simulink model "tilting_holocopter_approach"  (R2023b)
settings: Solver=VariableStepAuto  StartTime=0.0  StopTime=tot_time  RelTol=1e-3
InitFcn:
  | addpath('TRAJECTORIES\');
  | square_tilting
  | %circular_tilting
StartFcn:
  | %% Setup Video e Timer
  | videoFile = 'Holocopter_quad.avi';
  | %videoFile = 'Holocopter_circ.avi';
  | videoObj = VideoWriter(videoFile);
  | videoObj.FrameRate = 30;
  | open(videoObj);
  | assignin('base','videoObj',videoObj);
  | 
  | 
  | t = timer('ExecutionMode','fixedSpacing','Period',0.05,'StartDelay',2,...
  |           'TimerFcn',@(~,~) captureFrame(findall(0,'Type','figure','Name','UAV Animation'), videoObj));
  | start(t);
  | 
  | 
  | assignin('base','videoTimer',t);
StopFcn:
  | % Default graphics settings
  | set(0, 'DefaultTextInterpreter', 'latex')
  | set(0, 'DefaultLegendInterpreter', 'latex')
  | set(0, 'DefaultAxesTickLabelInterpreter', 'latex')
  | lw = 2;
  | plot_errors = figure('Renderer', 'painters', 'Position', [10 10 900 650]);
  | subplot(3,1,1)
  | plot(out.err_p.time, out.err_p.signals.values(1,:), 'k-', 'Linewidth', lw ,'Color', [0.2, 0.2, 0.2]);
  | hold on
  | plot(out.err_p.time, out.err_p.signals.values(2,:), 'k-', 'Linewidth', lw ,'Color', [1, 0, 0]);
  | hold on
  | plot(out.err_p.time, out.err_p.signals.values(3,:), 'k-', 'Linewidth', lw ,'Color', [0, 0, 1]);
  | legend({'x-axis', 'y-axis', 'z-axis'}, ...
  |        'Location', 'southeast', ...
  |        'Orientation', 'vertical', ...
  |        'FontSize', 12);
  | %xlabel('Time [s]')
  | ylabel('$e_p$ [m]')
  | set(gca, 'FontSize',18);
  | %Grid
  | grid on
  | box on
  | %----------------------------------------------------------
  | subplot(3,1,2)
  | plot(out.dot_err_p.time, out.dot_err_p.signals.values(1,:), 'k-', 'Linewidth', lw ,'Color', [0.2, 0.2, 0.2]);
  | hold on
  | plot(out.dot_err_p.time, out.dot_err_p.signals.values(2,:), 'k-', 'Linewidth', lw ,'Color', [1, 0, 0]);
  | hold on
  | plot(out.dot_err_p.time, out.dot_err_p.signals.values(3,:), 'k-', 'Linewidth', lw ,'Color', [0, 0, 1]);
  | legend({'x-axis', 'y-axis', 'z-axis'}, ...
  |        'Location', 'southeast', ...
  |        'Orientation', 'vertical', ...
  |        'FontSize', 12);
  | 
  | ylabel('$\dot{e}_p$ [m/s]')
  | set(gca, 'FontSize',18);
  | %Grid
  | grid on
  | box on
  | subplot(3,1,3)
  | plot(out.ddot_err_p.time, out.dot_err_p.signals.values(1,:), 'k-', 'Linewidth', lw ,'Color', [0.2, 0.2, 0.2]);
  | hold on
  | plot(out.ddot_err_p.time, out.dot_err_p.signals.values(2,:), 'k-', 'Linewidth', lw ,'Color', [1, 0, 0]);
  | hold on
  | plot(out.ddot_err_p.time, out.dot_err_p.signals.values(3,:), 'k-', 'Linewidth', lw ,'Color', [0, 0, 1]);
  | legend({'x-axis', 'y-axis', 'z-axis'}, ...
  |        'Location', 'southeast', ...
  |        'Orientation', 'vertical', ...
  |        'FontSize', 12);
  | xlabel('Time [s]')
  | ylabel('$\ddot{e}_p$ [m/$s^2$]')
  | set(gca, 'FontSize',18);
  | %Grid
  | grid on
  | box on
  | %Options
  | set(gcf,'color','w');
  | set(plot_errors, 'MenuBar', 'none', 'ToolBar', 'none');
  | exportgraphics(plot_errors, 'Tilting_holocopter_lin_err.pdf');
  | %--------------------------------------------------
  | plot_errors_or = figure('Renderer', 'painters', 'Position', [10 10 900 650]);
  | subplot(3,1,1)
  | plot(out.eR.time, out.eR.signals.values(1,:), 'k-', 'Linewidth', lw ,'Color', [0.2, 0.2, 0.2]);
  | hold on
  | plot(out.eR.time, out.eR.signals.values(2,:), 'k-', 'Linewidth', lw ,'Color', [1, 0, 0]);
  | hold on
  | plot(out.eR.time, out.eR.signals.values(3,:), 'k-', 'Linewidth', lw ,'Color', [0, 0, 1]);
  | legend({'x-axis', 'y-axis', 'z-axis'}, ...
  |        'Location', 'northeast', ...
  |        'Orientation', 'vertical', ...
  |        'FontSize', 10);
  | ylabel('$e_R$ [rad]')
  | set(gca, 'FontSize',18);
  | %Grid
  | grid on
  | box on
  | %----------------------------------------------------------
  | subplot(3,1,2)
  | plot(out.ew.time, out.ew.signals.values(1,:), 'k-', 'Linewidth', lw ,'Color', [0.2, 0.2, 0.2]);
  | hold on
  | plot(out.ew.time, out.ew.signals.values(2,:), 'k-', 'Linewidth', lw ,'Color', [1, 0, 0]);
  | hold on
  | plot(out.ew.time, out.ew.signals.values(3,:), 'k-', 'Linewidth', lw ,'Color', [0, 0, 1]);
  | legend({'x-axis', 'y-axis', 'z-axis'}, ...
  |        'Location', 'southeast', ...
  |        'Orientation', 'vertical', ...
  |        'FontSize', 10);
  | 
  | ylabel('$e_\omega$ [rad/s]')
  | set(gca, 'FontSize',18);
  | %Grid
  | grid on
  | box on
  | subplot(3,1,3)
  | plot(out.ea.time, out.ea.signals.values(1,:), 'k-', 'Linewidth', lw ,'Color', [0.2, 0.2, 0.2]);
  | hold on
  | plot(out.ea.time, out.ea.signals.values(2,:), 'k-', 'Linewidth', lw ,'Color', [1, 0, 0]);
  | hold on
  | plot(out.ea.time, out.ea.signals.values(3,:), 'k-', 'Linewidth', lw ,'Color', [0, 0, 1]);
  | legend({'x-axis', 'y-axis', 'z-axis'}, ...
  |        'Location', 'northeast', ...
  |        'Orientation', 'vertical', ...
  |        'FontSize', 8);
  | ylabel('$e_a$ [rad/$s^2$]')
  | xlabel('Time [s]')
  | set(gca, 'FontSize',18);
  | %Grid
  | grid on
  | box on
  | %Options
  | set(gcf,'color','w');
  | set(plot_errors_or, 'MenuBar', 'none', 'ToolBar', 'none');
  | exportgraphics(plot_errors_or, 'Tilting_holocopter_or_err.pdf');
  | %---------------------------------------------------------------------
  | 
  | 
  | 
  | %---------------------------------------------------------------------
  | 
  | 
  | videoObj = evalin('base','videoObj');
  | t = evalin('base','videoTimer');
  | 
  | 
  | stop(t);
  | delete(t);
  | close(videoObj);
  | 
  | 
  | clear videoObj videoTimer
  | disp('Saved Video UAV');
values from neighbouring files (symbols this model uses):
  cf = 1.65776*10^(-5)    (= 1.65776e-05)    [myConstraintsFcn.m]
  cm = 2.1792*10^(-7)    (= 2.1792e-07)    [myConstraintsFcn.m]
  l = 0.45    [myConstraintsFcn.m]
undefined symbols (not defined in the file or in its folder): Ib, lin_vel_0, mass, pos_0, Ts, w_bb_0
libraries: robotcorelib x1, matrix_library x1, uavutilslib x1
settings Model: Creator=fabioruggiero  LastModifiedBy=laura
settings ModelReferenceCC: EnableRefExpFcnMdlSchedulingChecks=on

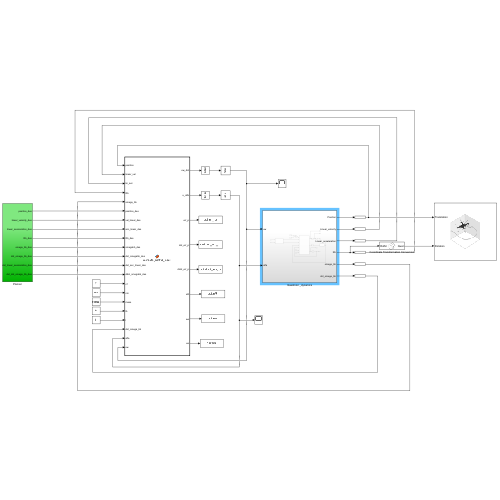
[thumbnail: Simulink's stored preview of the top-level diagram]
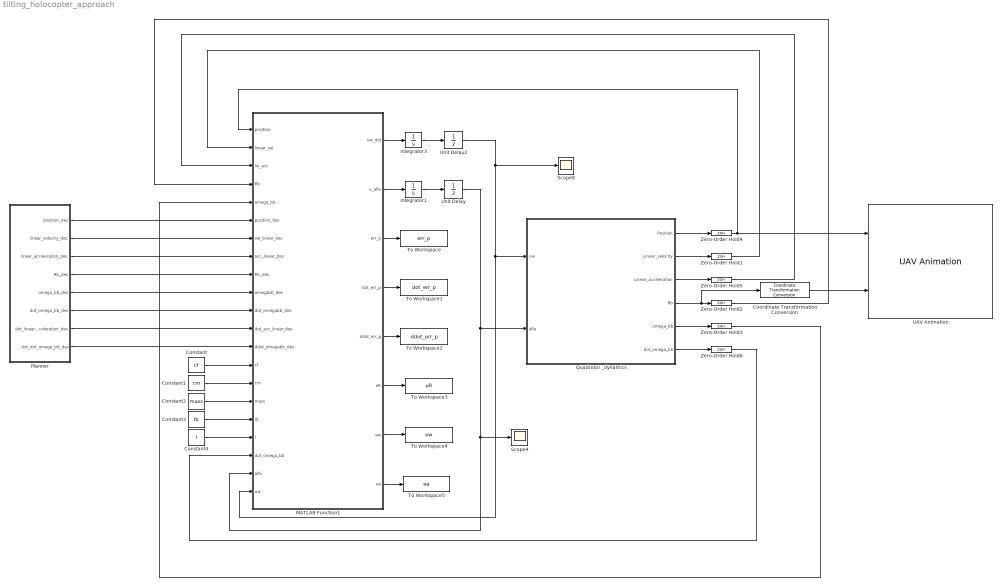
== system tilting_holocopter_approach ==
  Constant : Constant  Value=cf
  Constant1 : Constant  Value=cm
  Constant2 : Constant  Value=mass
  Constant3 : Constant  Value=Ib
  Constant4 : Constant  Value=l
  Coordinate Transformation Conversion : robotcorelib/Coordinate Transformation Conversion  InputRepresentation=Rotation Matrix  InputEulerSequence=ZYX  ShowTrVecInputPort=on  OutputRepresentation=Quaternion  OutputEulerSequence=ZYX  ShowTrVecOutputPort=on  SimulateUsing=Interpreted execution
  Integrator1 : Integrator  InitialCondition=[0.1 0.1 0.1 0.1]'
  Integrator3 : Integrator  InitialCondition=2e+05*ones(4,1)
  MATLAB Function1 : MATLAB Function  TreatAsAtomicUnit=on
  Planner : Subsystem
  Quadrotor _dynamics : Subsystem
  Scope4 : Scope
  Scope8 : Scope
  To Workspace : ToWorkspace  VariableName=err_p  SaveFormat=Structure With Time  SampleTime=-1
  To Workspace1 : ToWorkspace  VariableName=dot_err_p  SaveFormat=Structure With Time  SampleTime=-1
  To Workspace2 : ToWorkspace  VariableName=ddot_err_p  SaveFormat=Structure With Time  SampleTime=-1
  To Workspace3 : ToWorkspace  VariableName=eR  SaveFormat=Structure With Time  SampleTime=-1
  To Workspace4 : ToWorkspace  VariableName=ew  SaveFormat=Structure With Time  SampleTime=-1
  To Workspace5 : ToWorkspace  VariableName=ea  SaveFormat=Structure With Time  SampleTime=-1
  UAV Animation : uavutilslib/UAV Animation  UAVType=Multirotor  UAVSize=1  InertialZDirection=Down  SampleTime=0.01
  Unit Delay : UnitDelay  InitialCondition=[0.1 0.1 0.1 0.1]'  SampleTime=-1  HasFrameUpgradeWarning=on
  Unit Delay2 : UnitDelay  InitialCondition=2e+05*ones(4,1)  SampleTime=-1  HasFrameUpgradeWarning=on
  Zero-Order Hold{1..6} (6 alike) : ZeroOrderHold  SampleTime=Ts
  wires:
  Quadrotor _dynamics/1(Position) -> Zero-Order Hold4/1
  Quadrotor _dynamics/2(Linear_velocity) -> Zero-Order Hold1/1
  Quadrotor _dynamics/4(Rb) -> Coordinate Transformation Conversion/1, Zero-Order Hold2/1
  Quadrotor _dynamics/5(omega_bb) -> Zero-Order Hold3/1
  Zero-Order Hold4/1 -> UAV Animation/1, MATLAB Function1/1(position)
  Planner/1(position_des) -> MATLAB Function1/6(position_des)
  Coordinate Transformation Conversion/1 -> UAV Animation/2
  Quadrotor _dynamics/3(Linear_acceleration) -> Zero-Order Hold5/1
  Quadrotor _dynamics/6(dot_omega_bb) -> Zero-Order Hold6/1
  Planner/5(omega_bb_des) -> MATLAB Function1/10(omegabb_des)
  Planner/6(dot_omega_bb_des) -> MATLAB Function1/11(dot_omegabb_des)
  Zero-Order Hold5/1 -> MATLAB Function1/3(lin_acc)
  Zero-Order Hold1/1 -> MATLAB Function1/2(linear_vel)
  Zero-Order Hold3/1 -> MATLAB Function1/5(omega_bb)
  Zero-Order Hold2/1 -> MATLAB Function1/4(Rb)
  Planner/2(linear_velocity_des) -> MATLAB Function1/7(vel_linear_des)
  Planner/3(linear_acceleration_des) -> MATLAB Function1/8(acc_linear_des)
  Planner/4(Rb_des) -> MATLAB Function1/9(Rb_des)
  Constant/1 -> MATLAB Function1/14(cf)
  Constant1/1 -> MATLAB Function1/15(cm)
  Constant2/1 -> MATLAB Function1/16(mass)
  Constant3/1 -> MATLAB Function1/17(Ib)
  Constant4/1 -> MATLAB Function1/18(l)
  MATLAB Function1/1(uw_dot) -> Integrator3/1
  MATLAB Function1/6(eR) -> To Workspace3/1
  MATLAB Function1/7(ew) -> To Workspace4/1
  MATLAB Function1/3(err_p) -> To Workspace/1
  MATLAB Function1/4(dot_err_p) -> To Workspace1/1
  Zero-Order Hold6/1 -> MATLAB Function1/19(dot_omega_bb)
  Planner/7(dot_linear_acceleration_des) -> MATLAB Function1/12(dot_acc_linear_des)
  Planner/8(dot_dot_omega_bb_des) -> MATLAB Function1/13(ddot_omegabb_des)
  MATLAB Function1/2(u_alfa) -> Integrator1/1
  Unit Delay/1 -> Scope4/1, MATLAB Function1/20(alfa), Quadrotor _dynamics/2(alfa)
  Unit Delay2/1 -> MATLAB Function1/21(uw), Quadrotor _dynamics/1(uw), Scope8/1
  Integrator1/1 -> Unit Delay/1
  Integrator3/1 -> Unit Delay2/1
  MATLAB Function1/8(ea) -> To Workspace5/1
  MATLAB Function1/5(ddot_err_p) -> To Workspace2/1

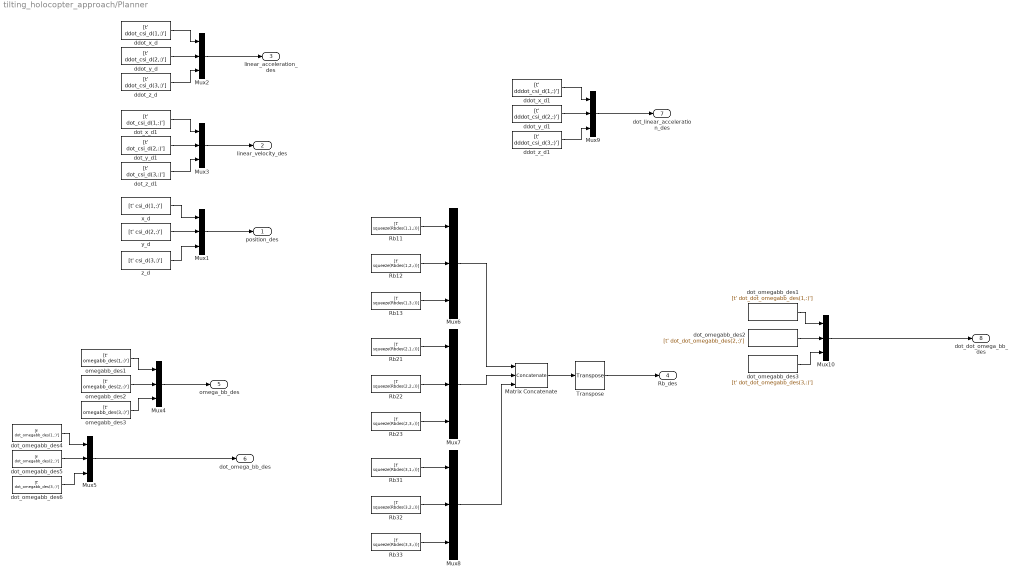
== system tilting_holocopter_approach/Planner ==
  Matrix Concatenate : Concatenate  NumInputs=3  Mode=Multidimensional array  ConcatenateDimension=2
  Mux{1..10} (10 alike) : Mux  Inputs=3
  Rb11 : FromWorkspace  VariableName=[t' squeeze(Rbdes(1,1,:))]  SampleTime=Ts
  Rb12 : FromWorkspace  VariableName=[t' squeeze(Rbdes(1,2,:))]  SampleTime=Ts
  Rb13 : FromWorkspace  VariableName=[t' squeeze(Rbdes(1,3,:))]  SampleTime=Ts
  Rb21 : FromWorkspace  VariableName=[t' squeeze(Rbdes(2,1,:))]  SampleTime=Ts
  Rb22 : FromWorkspace  VariableName=[t' squeeze(Rbdes(2,2,:))]  SampleTime=Ts
  Rb23 : FromWorkspace  VariableName=[t' squeeze(Rbdes(2,3,:))]  SampleTime=Ts
  Rb31 : FromWorkspace  VariableName=[t' squeeze(Rbdes(3,1,:))]  SampleTime=Ts
  Rb32 : FromWorkspace  VariableName=[t' squeeze(Rbdes(3,2,:))]  SampleTime=Ts
  Rb33 : FromWorkspace  VariableName=[t' squeeze(Rbdes(3,3,:))]  SampleTime=Ts
  Transpose : matrix_library/Transpose
  ddot_x_d : FromWorkspace  VariableName=[t' ddot_csi_d(1,:)']  SampleTime=Ts
  ddot_x_d1 : FromWorkspace  VariableName=[t' dddot_csi_d(1,:)']  SampleTime=Ts
  ddot_y_d : FromWorkspace  VariableName=[t' ddot_csi_d(2,:)']  SampleTime=Ts
  ddot_y_d1 : FromWorkspace  VariableName=[t' dddot_csi_d(2,:)']  SampleTime=Ts
  ddot_z_d : FromWorkspace  VariableName=[t' ddot_csi_d(3,:)']  SampleTime=Ts
  ddot_z_d1 : FromWorkspace  VariableName=[t' dddot_csi_d(3,:)']  SampleTime=Ts
  dot_omegabb_des1 : FromWorkspace  VariableName=[t' dot_dot_omegabb_des(1,:)']  SampleTime=Ts
  dot_omegabb_des2 : FromWorkspace  VariableName=[t' dot_dot_omegabb_des(2,:)']  SampleTime=Ts
  dot_omegabb_des3 : FromWorkspace  VariableName=[t' dot_dot_omegabb_des(3,:)']  SampleTime=Ts
  dot_omegabb_des4 : FromWorkspace  VariableName=[t' dot_omegabb_des(1,:)']  SampleTime=Ts
  dot_omegabb_des5 : FromWorkspace  VariableName=[t' dot_omegabb_des(2,:)']  SampleTime=Ts
  dot_omegabb_des6 : FromWorkspace  VariableName=[t' dot_omegabb_des(3,:)']  SampleTime=Ts
  dot_x_d1 : FromWorkspace  VariableName=[t' dot_csi_d(1,:)']  SampleTime=Ts
  dot_y_d1 : FromWorkspace  VariableName=[t' dot_csi_d(2,:)']  SampleTime=Ts
  dot_z_d1 : FromWorkspace  VariableName=[t' dot_csi_d(3,:)']  SampleTime=Ts
  omegabb_des1 : FromWorkspace  VariableName=[t' omegabb_des(1,:)']  SampleTime=Ts
  omegabb_des2 : FromWorkspace  VariableName=[t' omegabb_des(2,:)']  SampleTime=Ts
  omegabb_des3 : FromWorkspace  VariableName=[t' omegabb_des(3,:)']  SampleTime=Ts
  x_d : FromWorkspace  VariableName=[t' csi_d(1,:)']  SampleTime=Ts
  y_d : FromWorkspace  VariableName=[t' csi_d(2,:)']  SampleTime=Ts
  z_d : FromWorkspace  VariableName=[t' csi_d(3,:)']  SampleTime=Ts
  position_des : Outport
  linear_velocity_des : Outport  Port=2
  linear_acceleration_des : Outport  Port=3
  Rb_des : Outport  Port=4
  omega_bb_des : Outport  Port=5
  dot_omega_bb_des : Outport  Port=6
  dot_linear_acceleration_des : Outport  Port=7
  dot_dot_omega_bb_des : Outport  Port=8
  wires:
  y_d/1 -> Mux1/2
  z_d/1 -> Mux1/3
  x_d/1 -> Mux1/1
  ddot_y_d/1 -> Mux2/2
  ddot_z_d/1 -> Mux2/3
  ddot_x_d/1 -> Mux2/1
  Mux2/1 -> linear_acceleration_des/1
  Mux1/1 -> position_des/1
  dot_y_d1/1 -> Mux3/2
  dot_z_d1/1 -> Mux3/3
  dot_x_d1/1 -> Mux3/1
  Mux3/1 -> linear_velocity_des/1
  Mux5/1 -> dot_omega_bb_des/1
  omegabb_des3/1 -> Mux4/3
  Mux4/1 -> omega_bb_des/1
  omegabb_des2/1 -> Mux4/2
  omegabb_des1/1 -> Mux4/1
  dot_omegabb_des4/1 -> Mux5/1
  dot_omegabb_des5/1 -> Mux5/2
  dot_omegabb_des6/1 -> Mux5/3
  Rb11/1 -> Mux6/1
  Rb12/1 -> Mux6/2
  Rb13/1 -> Mux6/3
  Rb23/1 -> Mux7/3
  Rb22/1 -> Mux7/2
  Rb21/1 -> Mux7/1
  Rb31/1 -> Mux8/1
  Rb32/1 -> Mux8/2
  Rb33/1 -> Mux8/3
  Mux6/1 -> Matrix Concatenate/1
  Mux7/1 -> Matrix Concatenate/2
  Mux8/1 -> Matrix Concatenate/3
  Matrix Concatenate/1 -> Transpose/1
  Transpose/1 -> Rb_des/1
  Mux9/1 -> dot_linear_acceleration_des/1
  ddot_y_d1/1 -> Mux9/2
  ddot_z_d1/1 -> Mux9/3
  ddot_x_d1/1 -> Mux9/1
  dot_omegabb_des3/1 -> Mux10/3
  dot_omegabb_des1/1 -> Mux10/1
  dot_omegabb_des2/1 -> Mux10/2
  Mux10/1 -> dot_dot_omega_bb_des/1

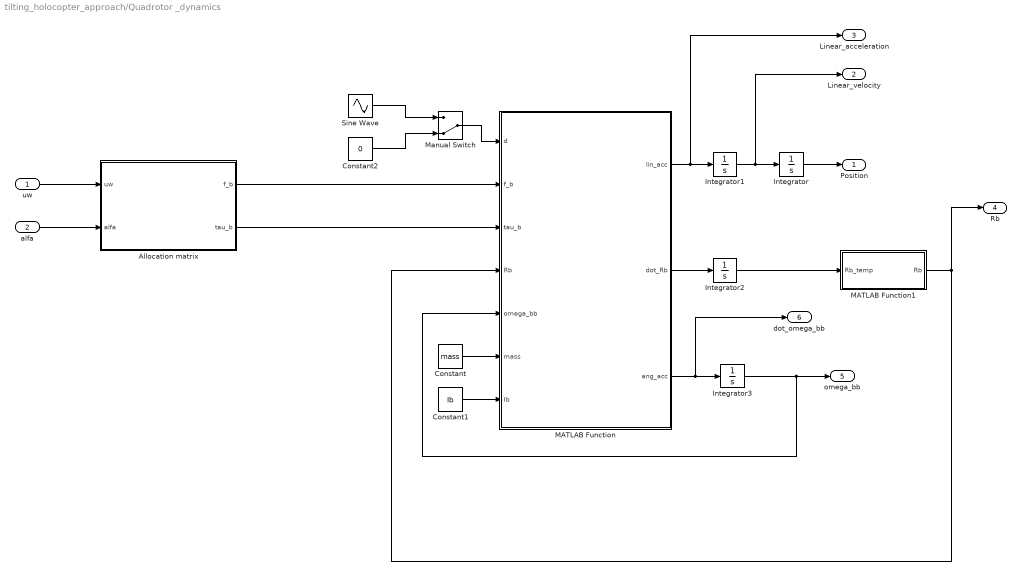
== system tilting_holocopter_approach/Quadrotor _dynamics ==
  uw : Inport
  alfa : Inport  Port=2
  Allocation matrix : MATLAB Function  TreatAsAtomicUnit=on
  Constant : Constant  Value=mass
  Constant1 : Constant  Value=Ib
  Constant2 : Constant  Value=0
  Integrator : Integrator  InitialCondition=pos_0'
  Integrator1 : Integrator  InitialCondition=lin_vel_0'
  Integrator2 : Integrator  InitialCondition=[1 0 0; 0 1 0;0 0 1]
  Integrator3 : Integrator  InitialCondition=w_bb_0'
  MATLAB Function : MATLAB Function  TreatAsAtomicUnit=on
  MATLAB Function1 : MATLAB Function  TreatAsAtomicUnit=on
  Manual Switch : ManualSwitch  CurrentSetting=0
  Sine Wave : Sin  Frequency=0.2  SampleTime=0
  Position : Outport
  Linear_velocity : Outport  Port=2
  Linear_acceleration : Outport  Port=3
  Rb : Outport  Port=4
  omega_bb : Outport  Port=5
  dot_omega_bb : Outport  Port=6
  wires:
  Integrator/1 -> Position/1
  MATLAB Function/3(ang_acc) -> dot_omega_bb/1, Integrator3/1
  Integrator1/1 -> Linear_velocity/1, Integrator/1
  Integrator3/1 -> omega_bb/1, MATLAB Function/5(omega_bb)
  MATLAB Function/2(dot_Rb) -> Integrator2/1
  MATLAB Function1/1(Rb) -> MATLAB Function/4(Rb), Rb/1
  Integrator2/1 -> MATLAB Function1/1(Rb_temp)
  Allocation matrix/1(f_b) -> MATLAB Function/2(f_b)
  Allocation matrix/2(tau_b) -> MATLAB Function/3(tau_b)
  MATLAB Function/1(lin_acc) -> Linear_acceleration/1, Integrator1/1
  Constant/1 -> MATLAB Function/6(mass)
  Constant1/1 -> MATLAB Function/7(Ib)
  uw/1 -> Allocation matrix/1(uw)
  alfa/1 -> Allocation matrix/2(alfa)
  Sine Wave/1 -> Manual Switch/1
  Constant2/1 -> Manual Switch/2
  Manual Switch/1 -> MATLAB Function/1(d)

== matlab function tilting_holocopter_approach/Quadrotor _dynamics/MATLAB Function1 ==
  data: Rb_temp input; Rb output
function Rb = fcn(Rb_temp)
    [U,S,V] = svd(Rb_temp);
    sigma = det(U*V');
    S_ = diag([1 1 sigma]);

    Rb = U*S_*V';
end

== matlab function tilting_holocopter_approach/Quadrotor _dynamics/Allocation matrix ==
  data: uw input size=4; alfa input size=4; f_b output size=3; tau_b output size=3; cm parameter; cf parameter; l parameter
function [f_b,tau_b] = allocation_matrix(uw,alfa,cm, cf, l)

alfa1 = alfa(1);
alfa2 = alfa(2);
alfa3 = alfa(3);
alfa4 = alfa(4);



Gq = [0 -cf*sin(alfa2) 0 cf*sin(alfa4);
      cf*sin(alfa1) 0 -cf*sin(alfa3) 0;
      -cf*cos(alfa1) -cf*cos(alfa2) -cf*cos(alfa3) -cf*cos(alfa4);
      0 -l*cf*cos(alfa2)-cm*sin(alfa2) 0 l*cf*cos(alfa4)+cm*sin(alfa4);
      l*cf*cos(alfa1)+cm*sin(alfa1) 0 -l*cf*cos(alfa3)-cm*sin(alfa3) 0;
      l*cf*sin(alfa1)-cm*cos(alfa1) -l*cf*sin(alfa2)+cm*cos(alfa2) l*cf*sin(alfa3)-cm*cos(alfa3) -l*cf*sin(alfa4)+cm*cos(alfa4)];


out = Gq*uw;
f_b = out(1:3);
tau_b = out(4:6);
end

== matlab function tilting_holocopter_approach/Quadrotor _dynamics/MATLAB Function ==
  data: d input; f_b input; lin_acc output; tau_b input; Rb input; omega_bb input; mass input; Ib input; dot_Rb output; ang_acc output
function [lin_acc, dot_Rb, ang_acc] = dynamics(d,f_b,tau_b,Rb,omega_bb,mass, Ib)

lin_acc = 9.81*[0 0 1]'+(1/mass)*Rb*f_b + d*ones(3,1);
dot_Rb = Rb*skew(omega_bb);
ang_acc = inv(Ib)*(-skew(omega_bb)*Ib*omega_bb + tau_b);


end

function S = skew(v)
if(numel(v)~= 1)
S= [0 -v(3) v(2); 
    v(3) 0 -v(1);
    -v(2) v(1) 0];
else
S= zeros(3);
end
end

== matlab function tilting_holocopter_approach/MATLAB Function1 ==
  data: position input; uw_dot output; linear_vel input; lin_acc input; Rb input; omega_bb input; position_des input; vel_linear_des input; acc_linear_des input; Rb_des input; omegabb_des input; dot_omegabb_des input; dot_acc_linear_des input; ddot_omegabb_des input; cf input; cm input; mass input; Ib input; l input; dot_omega_bb input; u_alfa output; err_p output; dot_err_p output; ddot_err_p output; eR output; ew output; alfa input; uw input; ea output
function [uw_dot, u_alfa, err_p, dot_err_p, ddot_err_p, eR, ew, ea] = compute_control_input(position, linear_vel, lin_acc, Rb, omega_bb, position_des, vel_linear_des, acc_linear_des, Rb_des, omegabb_des, dot_omegabb_des, ...
   dot_acc_linear_des, ddot_omegabb_des, cf, cm, mass, Ib, l,   dot_omega_bb,alfa,uw)

    %Compute errors
    err_p = position - position_des;
    dot_err_p = linear_vel - vel_linear_des;
    ddot_err_p = lin_acc - acc_linear_des; 
    eR = vee((Rb_des'*Rb - Rb'*Rb_des))/2;
    ew = omega_bb - Rb'*Rb_des*omegabb_des;
    ea = dot_omega_bb - Rb' * Rb_des * dot_omegabb_des;
    
    g = 9.81;
    
    alfa1 = alfa(1);
    alfa2 = alfa(2);
    alfa3 = alfa(3);
    alfa4 = alfa(4);
    
    uw1 = uw(1);
    uw2 = uw(2);
    uw3 = uw(3);
    uw4 = uw(4);
    
    %Allocation matrix
    Gq = [0 -cf*sin(alfa2) 0 cf*sin(alfa4);
        cf*sin(alfa1) 0 -cf*sin(alfa3) 0;
        -cf*cos(alfa1) -cf*cos(alfa2) -cf*cos(alfa3) -cf*cos(alfa4);
        0 -l*cf*cos(alfa2)-cm*sin(alfa2) 0 l*cf*cos(alfa4)+cm*sin(alfa4);
        l*cf*cos(alfa1)+cm*sin(alfa1) 0 -l*cf*cos(alfa3)-cm*sin(alfa3) 0;
        l*cf*sin(alfa1)-cm*cos(alfa1) -l*cf*sin(alfa2)+cm*cos(alfa2) l*cf*sin(alfa3)-cm*cos(alfa3) -l*cf*sin(alfa4)+cm*cos(alfa4)];
    
    %Gains
    k_pl = diag([50 50 100]);
    k_vl = diag([30 30 100]);
    k_al = diag([10 10 100]);
    k_pa = diag([4 4 4]);
    k_va = diag([sqrt(10) sqrt(10) sqrt(10)]);
    k_aa = diag([sqrt(sqrt(10)) sqrt(sqrt(10)) sqrt(sqrt(10))]);
    
    
    sum_part_d = [0 , -cf*cos(alfa2)*uw2 , 0 , cf*cos(alfa4)*uw4;
                  cf*cos(alfa1)*uw1 , 0 , -cf*cos(alfa3)*uw3 , 0;
                  cf*sin(alfa1)*uw1 , cf*sin(alfa2)*uw2 , cf*sin(alfa3)*uw3 , cf*sin(alfa4)*uw4;
                  0 , (l*cf*sin(alfa2)-cm*cos(alfa2))*uw2 , 0 , (-l*cf*sin(alfa4)+cm*cos(alfa4))*uw4;
                  (-l*cf*sin(alfa1)+cm*cos(alfa1))*uw1 , 0 , (l*cf*sin(alfa3)-cm*cos(alfa3))*uw3 , 0;
                  (l*cf*cos(alfa1)+cm*sin(alfa1))*uw1 , (-l*cf*cos(alfa2)-cm*sin(alfa2))*uw2 , (l*cf*cos(alfa3)+cm*sin(alfa3))*uw3 , (-l*cf*cos(alfa4)-cm*sin(alfa4))*uw4];
    
    A = inv([mass*eye(3) zeros(3);zeros(3) Ib])*[Rb zeros(3);zeros(3) eye(3)]*[Gq sum_part_d];
    b = inv([mass*eye(3) zeros(3);zeros(3) Ib])*([zeros(3,1);-skew(dot_omega_bb)*Ib*omega_bb-skew(omega_bb)*Ib*dot_omega_bb]+[Rb*skew(omega_bb) zeros(3);zeros(3) zeros(3)]*Gq*uw);
    
    %Virtual input for the feedback linearization
    v = [-k_pl*err_p-k_vl*dot_err_p-k_al*ddot_err_p+dot_acc_linear_des; -k_pa*eR-k_va*ew-k_aa*ea+ddot_omegabb_des];

    %Conmpute control input 
    control_input = pinv(A)*(v-b);
    uw_dot = control_input(1:4);
    u_alfa = control_input(5:8);


end

function S = skew(v)
if(numel(v)~= 1)
S= [0 -v(3) v(2); 
    v(3) 0 -v(1);
    -v(2) v(1) 0];
else
S= zeros(3);
end
end

function v = vee(S)
v = [S(3,2); S(1,3); S(2,1)];
end
